simulink model "blown_wing_model"  (R2026a)
settings: Solver=ode23  StopTime=1000  MaxStep=0.05
InitFcn:
  | init_params
values from neighbouring files (symbols this model uses):
  alpha_deg_grid = params.alpha_deg_grid    [init_params.m]
  b = params.b    [init_params.m]
  c = params.c    [init_params.m]    (also in run_aa222_opt.m = clReqProxy - 0.98 * max(params.cl_all_high_lift))
  c_ht = params.c_ht    [init_params.m]
  cd_all_high_lift = params.cd_all_high_lift    [init_params.m]
  cd_blow_only = params.cd_blow_only    [init_params.m]
  cd_clean_baseline = params.cd_clean_baseline    [init_params.m]
  cd_flap_only = params.cd_flap_only    [init_params.m]
  cg_x_m = params.cg_x_m    [init_params.m]
  cl_all_high_lift = params.cl_all_high_lift    [init_params.m]
  CL_alpha_ht = params.CL_alpha_ht    [init_params.m]
  cl_blow_only = params.cl_blow_only    [init_params.m]
  cl_clean_baseline = params.cl_clean_baseline    [init_params.m]
  CL_delta_e = params.CL_delta_e    [init_params.m]
  cl_flap_only = params.cl_flap_only    [init_params.m]
  cm_all_high_lift = params.cm_all_high_lift    [init_params.m]
  cm_blow_only = params.cm_blow_only    [init_params.m]
  cm_clean_baseline = params.cm_clean_baseline    [init_params.m]
  cm_flap_only = params.cm_flap_only    [init_params.m]
  D_prop = params.D_prop    [init_params.m]
  flap_deflection_slow = params.flap_deflection_slow    [init_params.m]
  flap_span_fraction = params.flap_span_fraction    [init_params.m]
  k_span_expansion = params.k_span_expansion    [init_params.m]
  lt = params.lt    [init_params.m]
  params = struct()    [aa222_load_capstone_config.m]    (also in compute_cost.m = aa222_load_capstone_config(fullfile(pwd, 'AA146-Capstone')); init_params.m = aa222_load_capstone_config(capstoneRoot))
  prop_axial_x_m = params.prop_axial_x_m    [init_params.m]
  prop_rpm_grid = params.prop_rpm_grid    [init_params.m]
  prop_thrust_grid = params.prop_thrust_grid    [init_params.m]
  S_ht = params.S_ht    [init_params.m]
  y_dist = params.y_dist    [init_params.m]
libraries: aerolibobsolete x1, aerolibatmos2 x1
settings Model: Creator=olinw  LastModifiedBy=olinw
settings DataIOCC: ExternalInput=utest

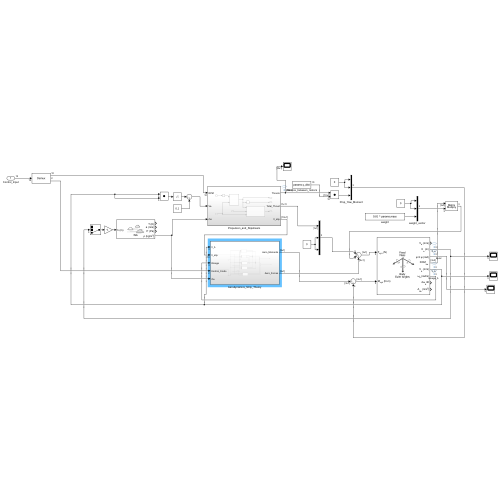
[thumbnail: Simulink's stored preview of the top-level diagram]
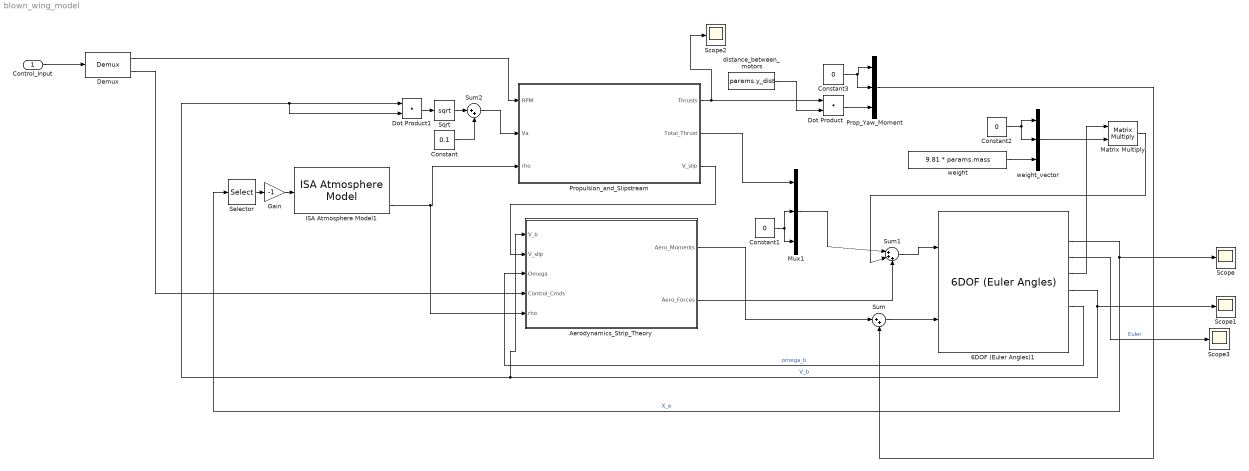
== system blown_wing_model ==
  Control_Input : Inport  PortDimensions=12
  6DOF (Euler Angles)1 : aerolibobsolete/6DOF (Euler Angles)  units=Metric (MKS)  mtype=Fixed  rep=Euler Angles  xme_0=initial_pos_ned  Vm_0=initial_vel_body  eul_0=[0 0 0]  pm_0=[0 0 0]  mass_0=params.mass  mass_e=0.5  mass_f=2.0  inertia=params.InertiaMatrix  inertia_e=eye(3)  inertia_f=2*eye(3)  k_quat=1.0  vre_flag=on  abi_flag=off  aMode=0  xme_statename=''  Vm_statename=''  eul_statename=''  quat_statename=''  pm_statename=''  mass_statename=''
  Aerodynamics_Strip_Theory : Subsystem
  Constant : Constant  Value=0.1
  Constant1 : Constant  Value=0
  Constant2 : Constant  Value=0
  Constant3 : Constant  Value=0
  Demux : Demux  Outputs=[10 2]
      settings: DisplayOption=none
  Dot Product : DotProduct  OutDataTypeStr=Inherit: Inherit via internal rule
  Dot Product1 : DotProduct  OutDataTypeStr=Inherit: Inherit via internal rule
  Gain : Gain  Gain=-1
  ISA Atmosphere Model1 : aerolibatmos2/ISA Atmosphere Model  useExtended=off  action=None  custom=off  viscosityOut=off  g=9.80665  gamma=1.4  R=287.0531  L=0.0065  h_trop=11000  h_strat=20000  rho0=1.225  P0=101325  T0=288.15  h0=0  S=110.4  Tref=273.15  muref=1.716e-5
  Matrix Multiply : Product  Multiplication=Matrix(*)
  Mux1 : Mux  Inputs=3
  Prop_Yaw_Moment : Mux  Inputs=3
  Propulsion_and_Slipstream : Subsystem
  Scope{,1..3} (4 alike) : Scope
      Scope settings: ActiveDisplayYMinimum=-13352.639774194251  ActiveDisplayYMaximum=3591.5339241802285
      Scope1 settings: ActiveDisplayYMinimum=-4.7629764478395824  ActiveDisplayYMaximum=24.22748883276633
      Scope2 settings: ActiveDisplayYMinimum=0.086325999999999986  ActiveDisplayYMaximum=0.28632599999999997  DataLoggingVariableName=ScopeData2
      Scope3 settings: ActiveDisplayYMinimum=-3.92486986686931  ActiveDisplayYMaximum=3.9215936057771783  DataLoggingVariableName=ScopeData3
  Selector : Selector  InputPortWidth=3  IndexOptions=Index vector (dialog)  Indices=3  OutputSizes=1
  Sqrt : Sqrt
  Sum : Sum  Inputs=|++
  Sum1 : Sum  Inputs=|+++
  Sum2 : Sum  Inputs=|++
  distance_between_motors : Constant  Value=params.y_dist
  weight : Constant  Value=9.81 * params.mass
  weight_vector : Mux  Inputs=3
  wires:
  Propulsion_and_Slipstream/2(Total_Thrust) -> Mux1/1
  Constant1/1 -> Mux1/3, Mux1/2
  weight_vector/1 -> Matrix Multiply/2
  Sum1/1 -> 6DOF (Euler Angles)1/1
  6DOF (Euler Angles)1/2 -> Scope/1, Selector/1  "X_e"
  ISA Atmosphere Model1/4 -> Aerodynamics_Strip_Theory/5(rho), Propulsion_and_Slipstream/3(rho)
  6DOF (Euler Angles)1/5 -> Scope1/1, Aerodynamics_Strip_Theory/1(V_b), Dot Product1/2, Dot Product1/1  "V_b"
  Propulsion_and_Slipstream/3(V_slip) -> Aerodynamics_Strip_Theory/2(V_slip)
  Mux1/1 -> Sum1/1
  Aerodynamics_Strip_Theory/2(Aero_Forces) -> Sum1/3
  weight/1 -> weight_vector/3
  distance_between_motors/1 -> Dot Product/2
  Propulsion_and_Slipstream/1(Thrusts) -> Scope2/1, Dot Product/1
  Dot Product/1 -> Prop_Yaw_Moment/3
  Constant3/1 -> Prop_Yaw_Moment/2, Prop_Yaw_Moment/1
  Prop_Yaw_Moment/1 -> Sum/2
  Aerodynamics_Strip_Theory/1(Aero_Moments) -> Sum/1
  Sum/1 -> 6DOF (Euler Angles)1/2
  Constant2/1 -> weight_vector/2, weight_vector/1
  Selector/1 -> Gain/1
  Gain/1 -> ISA Atmosphere Model1/1
  Dot Product1/1 -> Sqrt/1
  Sqrt/1 -> Sum2/1
  Constant/1 -> Sum2/2
  Sum2/1 -> Propulsion_and_Slipstream/2(Va)
  6DOF (Euler Angles)1/4 -> Matrix Multiply/1
  Matrix Multiply/1 -> Sum1/2
  Control_Input/1 -> Demux/1
  6DOF (Euler Angles)1/6 -> Aerodynamics_Strip_Theory/3(Omega)  "omega_b"
  Demux/1 -> Propulsion_and_Slipstream/1(RPM)
  Demux/2 -> Aerodynamics_Strip_Theory/4(Control_Cmds)
  6DOF (Euler Angles)1/3 -> Scope3/1  "Euler"

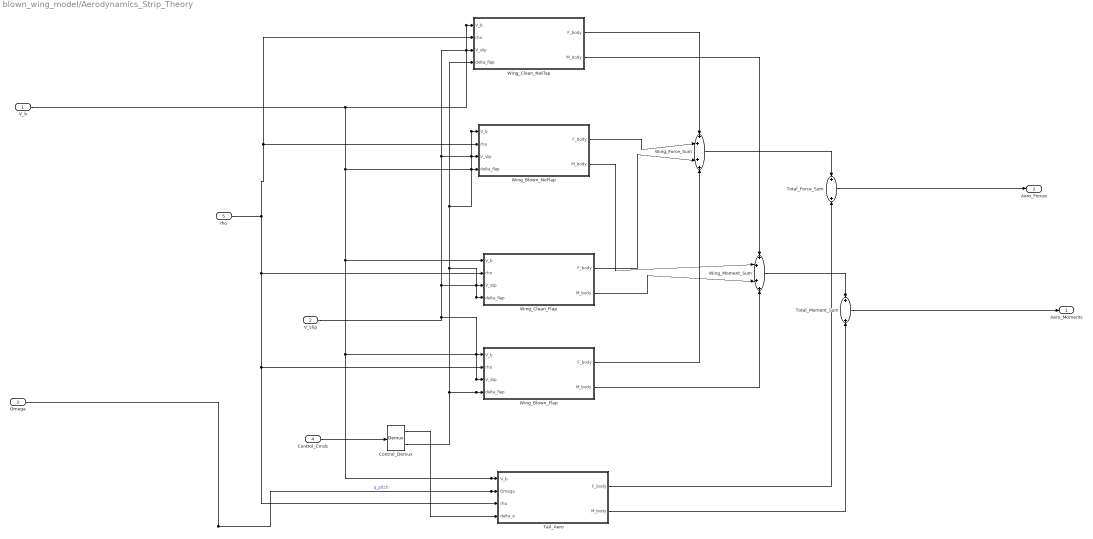
== system blown_wing_model/Aerodynamics_Strip_Theory ==
  V_b : Inport  PortDimensions=3
  V_slip : Inport  Port=2  PortDimensions=10
  Omega : Inport  Port=3
  Control_Cmds : Inport  Port=4
  rho : Inport  Port=5
  Control_Demux : Demux  Outputs=2
  Tail_Aero : Subsystem
  Total_Force_Sum : Sum
  Total_Moment_Sum : Sum
  Wing_Blown_Flap : Subsystem
  Wing_Blown_NoFlap : Subsystem
  Wing_Clean_Flap : Subsystem
  Wing_Clean_NoFlap : Subsystem
  Wing_Force_Sum : Sum  Inputs=++++
  Wing_Moment_Sum : Sum  Inputs=++++
  Aero_Moments : Outport
  Aero_Forces : Outport  Port=2
  wires:
  V_b/1 -> Tail_Aero/1(V_b), Wing_Blown_Flap/1(V_b), Wing_Clean_Flap/1(V_b), Wing_Blown_NoFlap/1(V_b), Wing_Clean_NoFlap/1(V_b)
  V_slip/1 -> Wing_Blown_Flap/3(V_slip), Wing_Blown_NoFlap/3(V_slip), Wing_Clean_NoFlap/3(V_slip), Wing_Clean_Flap/3(V_slip)
  Omega/1 -> Tail_Aero/2(Omega)  "q_pitch"
  Control_Cmds/1 -> Control_Demux/1
  Control_Demux/2 -> Wing_Blown_NoFlap/4(delta_flap), Wing_Clean_NoFlap/4(delta_flap), Wing_Clean_Flap/4(delta_flap), Wing_Blown_Flap/4(delta_flap)
  Control_Demux/1 -> Tail_Aero/4(delta_e)
  Wing_Force_Sum/1 -> Total_Force_Sum/1
  Wing_Moment_Sum/1 -> Total_Moment_Sum/1
  Total_Force_Sum/1 -> Aero_Forces/1
  Total_Moment_Sum/1 -> Aero_Moments/1
  Wing_Clean_NoFlap/1(F_body) -> Wing_Force_Sum/1
  Wing_Clean_NoFlap/2(M_body) -> Wing_Moment_Sum/1
  Wing_Blown_NoFlap/1(F_body) -> Wing_Force_Sum/2
  Wing_Blown_NoFlap/2(M_body) -> Wing_Moment_Sum/2
  Wing_Clean_Flap/1(F_body) -> Wing_Force_Sum/3
  Wing_Clean_Flap/2(M_body) -> Wing_Moment_Sum/3
  Wing_Blown_Flap/1(F_body) -> Wing_Force_Sum/4
  Wing_Blown_Flap/2(M_body) -> Wing_Moment_Sum/4
  Tail_Aero/2(M_body) -> Total_Moment_Sum/2
  Tail_Aero/1(F_body) -> Total_Force_Sum/2
  rho/1 -> Wing_Clean_Flap/2(rho), Tail_Aero/3(rho), Wing_Blown_Flap/2(rho), Wing_Clean_NoFlap/2(rho), Wing_Blown_NoFlap/2(rho)

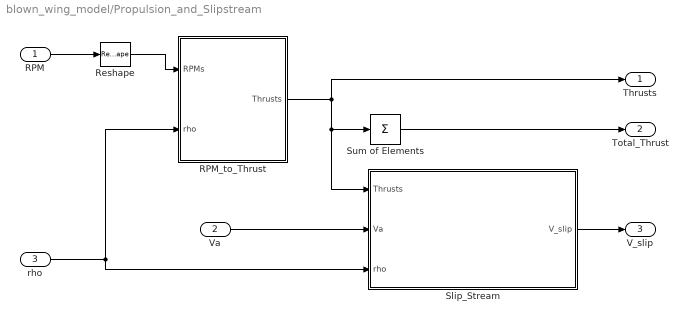
== system blown_wing_model/Propulsion_and_Slipstream ==
  RPM : Inport
  Va : Inport  Port=2
  rho : Inport  Port=3
  RPM_to_Thrust : MATLAB Function  TreatAsAtomicUnit=on
  Reshape : Reshape  OutputDimensionality=Customize  OutputDimensions=[10 1]
  Slip_Stream : MATLAB Function  TreatAsAtomicUnit=on
  Sum of Elements : Sum  Inputs=+
  Thrusts : Outport
  Total_Thrust : Outport  Port=2
  V_slip : Outport  Port=3
  wires:
  RPM_to_Thrust/1(Thrusts) -> Thrusts/1, Slip_Stream/1(Thrusts), Sum of Elements/1
  Sum of Elements/1 -> Total_Thrust/1
  Va/1 -> Slip_Stream/2(Va)
  rho/1 -> RPM_to_Thrust/2(rho), Slip_Stream/3(rho)
  Slip_Stream/1(V_slip) -> V_slip/1
  RPM/1 -> Reshape/1
  Reshape/1 -> RPM_to_Thrust/1(RPMs)

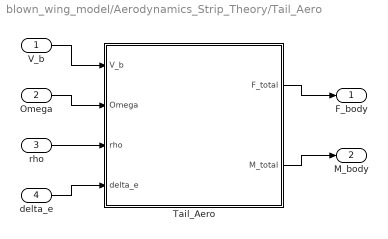
== system blown_wing_model/Aerodynamics_Strip_Theory/Tail_Aero ==
  V_b : Inport
  Omega : Inport  Port=2
  rho : Inport  Port=3
  delta_e : Inport  Port=4
  Tail_Aero : MATLAB Function  TreatAsAtomicUnit=on
  F_body : Outport
  M_body : Outport  Port=2
  wires:
  V_b/1 -> Tail_Aero/1(V_b)
  Omega/1 -> Tail_Aero/2(Omega)
  rho/1 -> Tail_Aero/3(rho)
  delta_e/1 -> Tail_Aero/4(delta_e)
  Tail_Aero/1(F_total) -> F_body/1
  Tail_Aero/2(M_total) -> M_body/1

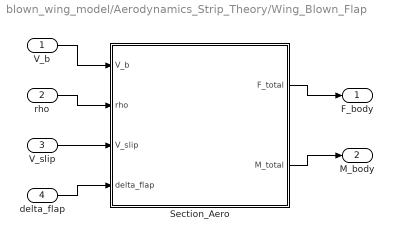
== system blown_wing_model/Aerodynamics_Strip_Theory/Wing_Blown_Flap ==
  V_b : Inport
  rho : Inport  Port=2
  V_slip : Inport  Port=3
  delta_flap : Inport  Port=4
  Section_Aero : MATLAB Function  TreatAsAtomicUnit=on
  F_body : Outport
  M_body : Outport  Port=2
  wires:
  V_b/1 -> Section_Aero/1(V_b)
  rho/1 -> Section_Aero/2(rho)
  V_slip/1 -> Section_Aero/3(V_slip)
  delta_flap/1 -> Section_Aero/4(delta_flap)
  Section_Aero/1(F_total) -> F_body/1
  Section_Aero/2(M_total) -> M_body/1

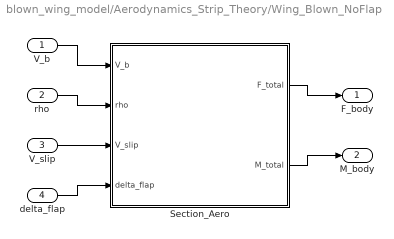
== system blown_wing_model/Aerodynamics_Strip_Theory/Wing_Blown_NoFlap ==
  V_b : Inport
  rho : Inport  Port=2
  V_slip : Inport  Port=3
  delta_flap : Inport  Port=4
  Section_Aero : MATLAB Function  TreatAsAtomicUnit=on
  F_body : Outport
  M_body : Outport  Port=2
  wires:
  V_b/1 -> Section_Aero/1(V_b)
  rho/1 -> Section_Aero/2(rho)
  V_slip/1 -> Section_Aero/3(V_slip)
  delta_flap/1 -> Section_Aero/4(delta_flap)
  Section_Aero/1(F_total) -> F_body/1
  Section_Aero/2(M_total) -> M_body/1

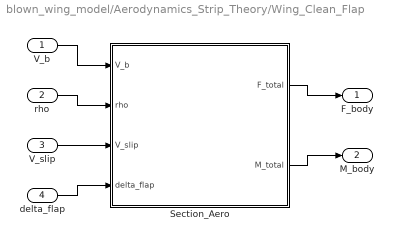
== system blown_wing_model/Aerodynamics_Strip_Theory/Wing_Clean_Flap ==
  V_b : Inport
  rho : Inport  Port=2
  V_slip : Inport  Port=3
  delta_flap : Inport  Port=4
  Section_Aero : MATLAB Function  TreatAsAtomicUnit=on
  F_body : Outport
  M_body : Outport  Port=2
  wires:
  V_b/1 -> Section_Aero/1(V_b)
  rho/1 -> Section_Aero/2(rho)
  V_slip/1 -> Section_Aero/3(V_slip)
  delta_flap/1 -> Section_Aero/4(delta_flap)
  Section_Aero/1(F_total) -> F_body/1
  Section_Aero/2(M_total) -> M_body/1

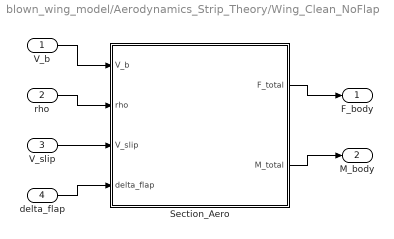
== system blown_wing_model/Aerodynamics_Strip_Theory/Wing_Clean_NoFlap ==
  V_b : Inport
  rho : Inport  Port=2
  V_slip : Inport  Port=3
  delta_flap : Inport  Port=4
  Section_Aero : MATLAB Function  TreatAsAtomicUnit=on
  F_body : Outport
  M_body : Outport  Port=2
  wires:
  V_b/1 -> Section_Aero/1(V_b)
  rho/1 -> Section_Aero/2(rho)
  V_slip/1 -> Section_Aero/3(V_slip)
  delta_flap/1 -> Section_Aero/4(delta_flap)
  Section_Aero/1(F_total) -> F_body/1
  Section_Aero/2(M_total) -> M_body/1

== matlab function blown_wing_model/Aerodynamics_Strip_Theory/Wing_Clean_Flap/Section_Aero ==
  data: V_b input; F_total output; rho input; V_slip input; delta_flap input; M_total output; y_dist parameter; D_prop parameter; b parameter; c parameter; cg_x_m parameter; prop_axial_x_m parameter; flap_span_fraction parameter; flap_deflection_slow parameter; k_span_expansion parameter; alpha_deg_grid parameter; cl_clean_baseline parameter; cl_blow_only parameter; cl_flap_only parameter; cl_all_high_lift parameter; cd_clean_baseline parameter; cd_blow_only parameter; cd_flap_only parameter; cd_all_high_lift parameter; cm_clean_baseline parameter; cm_blow_only parameter; cm_flap_only parameter; cm_all_high_lift parameter
function [F_total, M_total] = Section_Aero(V_b, rho, V_slip, delta_flap, y_dist, D_prop, b, c, cg_x_m, prop_axial_x_m, flap_span_fraction, flap_deflection_slow, k_span_expansion, alpha_deg_grid, cl_clean_baseline, cl_blow_only, cl_flap_only, cl_all_high_lift, cd_clean_baseline, cd_blow_only, cd_flap_only, cd_all_high_lift, cm_clean_baseline, cm_blow_only, cm_flap_only, cm_all_high_lift)
wantBlown = 0;
wantFlap = 1;
F_total = zeros(3,1);
M_total = zeros(3,1);
Vb = reshape(V_b, 3, 1);
Vsl = V_slip(:);
u = Vb(1);
w = Vb(3);
Va = sqrt(sum(Vb.^2)) + 1.0e-3;
alpha = atan2(w, u);
alphaDeg = alpha * 180.0 / pi;
qInf = 0.5 * rho * Va^2;
posMask = y_dist(:) > 0;
posCenters = y_dist(posMask);
posSlip = Vsl(posMask);
blownHalfWidth = 0.5 * k_span_expansion * D_prop;
semiSpan = 0.5 * b;
flapEnd = flap_span_fraction * semiSpan;
edgeList = [0; flapEnd; semiSpan; max(posCenters - blownHalfWidth, 0); min(posCenters + blownHalfWidth, semiSpan)];
edgeList = sort(unique(edgeList));
flapMix = min(max(abs(delta_flap) / max(flap_deflection_slow, 1.0e-6), 0), 1);
ca = cos(alpha);
sa = sin(alpha);
Rsb = [ca, 0, -sa; 0, 1, 0; sa, 0, ca];
for i = 1:(numel(edgeList) - 1)
    y0 = edgeList(i);
    y1 = edgeList(i + 1);
    width = y1 - y0;
    if width <= 1.0e-6
        continue;
    end
    yMid = 0.5 * (y0 + y1);
    isFlapRegion = (yMid <= flapEnd + 1.0e-9);
    overlapMask = (posCenters + blownHalfWidth > y0) & (posCenters - blownHalfWidth < y1);
    isBlownRegion = any(overlapMask);
    if isFlapRegion ~= wantFlap || isBlownRegion ~= wantBlown
        continue;
    end
    qLocal = qInf;
    if isBlownRegion
        vLocal = mean(posSlip(overlapMask));
        qLocal = 0.5 * rho * vLocal^2;
    end
    if wantBlown
        clNoFlap = interp1(alpha_deg_grid, cl_blow_only, alphaDeg, 'linear', 'extrap');
        cdNoFlap = interp1(alpha_deg_grid, cd_blow_only, alphaDeg, 'linear', 'extrap');
        cmNoFlap = interp1(alpha_deg_grid, cm_blow_only, alphaDeg, 'linear', 'extrap');
        clFlap = interp1(alpha_deg_grid, cl_all_high_lift, alphaDeg, 'linear', 'extrap');
        cdFlap = interp1(alpha_deg_grid, cd_all_high_lift, alphaDeg, 'linear', 'extrap');
        cmFlap = interp1(alpha_deg_grid, cm_all_high_lift, alphaDeg, 'linear', 'extrap');
    else
        clNoFlap = interp1(alpha_deg_grid, cl_clean_baseline, alphaDeg, 'linear', 'extrap');
        cdNoFlap = interp1(alpha_deg_grid, cd_clean_baseline, alphaDeg, 'linear', 'extrap');
        cmNoFlap = interp1(alpha_deg_grid, cm_clean_baseline, alphaDeg, 'linear', 'extrap');
        clFlap = interp1(alpha_deg_grid, cl_flap_only, alphaDeg, 'linear', 'extrap');
        cdFlap = interp1(alpha_deg_grid, cd_flap_only, alphaDeg, 'linear', 'extrap');
        cmFlap = interp1(alpha_deg_grid, cm_flap_only, alphaDeg, 'linear', 'extrap');
    end
    if wantFlap
        CL = clNoFlap + flapMix * (clFlap - clNoFlap);
        CD = cdNoFlap + flapMix * (cdFlap - cdNoFlap);
        Cm = cmNoFlap + flapMix * (cmFlap - cmNoFlap);
    else
        CL = clNoFlap;
        CD = cdNoFlap;
        Cm = cmNoFlap;
    end
    areaStrip = c * width;
    Fstab = qLocal * areaStrip * [-CD; 0; -CL];
    Fbody = Rsb * Fstab;
    Maero = qLocal * areaStrip * [0; Cm * c; 0];
    y = yMid;
    rVec = [prop_axial_x_m - cg_x_m; y; 0];
    Mlever = cross(rVec, Fbody);
    F_total = F_total + Fbody;
    M_total = M_total + Maero + Mlever;
    y = -yMid;
    rVec = [prop_axial_x_m - cg_x_m; y; 0];
    Mlever = cross(rVec, Fbody);
    F_total = F_total + Fbody;
    M_total = M_total + Maero + Mlever;
end
end

== matlab function blown_wing_model/Aerodynamics_Strip_Theory/Wing_Blown_Flap/Section_Aero ==
  data: V_b input; F_total output; rho input; V_slip input; delta_flap input; M_total output; y_dist parameter; D_prop parameter; b parameter; c parameter; cg_x_m parameter; prop_axial_x_m parameter; flap_span_fraction parameter; flap_deflection_slow parameter; k_span_expansion parameter; alpha_deg_grid parameter; cl_clean_baseline parameter; cl_blow_only parameter; cl_flap_only parameter; cl_all_high_lift parameter; cd_clean_baseline parameter; cd_blow_only parameter; cd_flap_only parameter; cd_all_high_lift parameter; cm_clean_baseline parameter; cm_blow_only parameter; cm_flap_only parameter; cm_all_high_lift parameter
function [F_total, M_total] = Section_Aero(V_b, rho, V_slip, delta_flap, y_dist, D_prop, b, c, cg_x_m, prop_axial_x_m, flap_span_fraction, flap_deflection_slow, k_span_expansion, alpha_deg_grid, cl_clean_baseline, cl_blow_only, cl_flap_only, cl_all_high_lift, cd_clean_baseline, cd_blow_only, cd_flap_only, cd_all_high_lift, cm_clean_baseline, cm_blow_only, cm_flap_only, cm_all_high_lift)
wantBlown = 1;
wantFlap = 1;
F_total = zeros(3,1);
M_total = zeros(3,1);
Vb = reshape(V_b, 3, 1);
Vsl = V_slip(:);
u = Vb(1);
w = Vb(3);
Va = sqrt(sum(Vb.^2)) + 1.0e-3;
alpha = atan2(w, u);
alphaDeg = alpha * 180.0 / pi;
qInf = 0.5 * rho * Va^2;
posMask = y_dist(:) > 0;
posCenters = y_dist(posMask);
posSlip = Vsl(posMask);
blownHalfWidth = 0.5 * k_span_expansion * D_prop;
semiSpan = 0.5 * b;
flapEnd = flap_span_fraction * semiSpan;
edgeList = [0; flapEnd; semiSpan; max(posCenters - blownHalfWidth, 0); min(posCenters + blownHalfWidth, semiSpan)];
edgeList = sort(unique(edgeList));
flapMix = min(max(abs(delta_flap) / max(flap_deflection_slow, 1.0e-6), 0), 1);
ca = cos(alpha);
sa = sin(alpha);
Rsb = [ca, 0, -sa; 0, 1, 0; sa, 0, ca];
for i = 1:(numel(edgeList) - 1)
    y0 = edgeList(i);
    y1 = edgeList(i + 1);
    width = y1 - y0;
    if width <= 1.0e-6
        continue;
    end
    yMid = 0.5 * (y0 + y1);
    isFlapRegion = (yMid <= flapEnd + 1.0e-9);
    overlapMask = (posCenters + blownHalfWidth > y0) & (posCenters - blownHalfWidth < y1);
    isBlownRegion = any(overlapMask);
    if isFlapRegion ~= wantFlap || isBlownRegion ~= wantBlown
        continue;
    end
    qLocal = qInf;
    if isBlownRegion
        vLocal = mean(posSlip(overlapMask));
        qLocal = 0.5 * rho * vLocal^2;
    end
    if wantBlown
        clNoFlap = interp1(alpha_deg_grid, cl_blow_only, alphaDeg, 'linear', 'extrap');
        cdNoFlap = interp1(alpha_deg_grid, cd_blow_only, alphaDeg, 'linear', 'extrap');
        cmNoFlap = interp1(alpha_deg_grid, cm_blow_only, alphaDeg, 'linear', 'extrap');
        clFlap = interp1(alpha_deg_grid, cl_all_high_lift, alphaDeg, 'linear', 'extrap');
        cdFlap = interp1(alpha_deg_grid, cd_all_high_lift, alphaDeg, 'linear', 'extrap');
        cmFlap = interp1(alpha_deg_grid, cm_all_high_lift, alphaDeg, 'linear', 'extrap');
    else
        clNoFlap = interp1(alpha_deg_grid, cl_clean_baseline, alphaDeg, 'linear', 'extrap');
        cdNoFlap = interp1(alpha_deg_grid, cd_clean_baseline, alphaDeg, 'linear', 'extrap');
        cmNoFlap = interp1(alpha_deg_grid, cm_clean_baseline, alphaDeg, 'linear', 'extrap');
        clFlap = interp1(alpha_deg_grid, cl_flap_only, alphaDeg, 'linear', 'extrap');
        cdFlap = interp1(alpha_deg_grid, cd_flap_only, alphaDeg, 'linear', 'extrap');
        cmFlap = interp1(alpha_deg_grid, cm_flap_only, alphaDeg, 'linear', 'extrap');
    end
    if wantFlap
        CL = clNoFlap + flapMix * (clFlap - clNoFlap);
        CD = cdNoFlap + flapMix * (cdFlap - cdNoFlap);
        Cm = cmNoFlap + flapMix * (cmFlap - cmNoFlap);
    else
        CL = clNoFlap;
        CD = cdNoFlap;
        Cm = cmNoFlap;
    end
    areaStrip = c * width;
    Fstab = qLocal * areaStrip * [-CD; 0; -CL];
    Fbody = Rsb * Fstab;
    Maero = qLocal * areaStrip * [0; Cm * c; 0];
    y = yMid;
    rVec = [prop_axial_x_m - cg_x_m; y; 0];
    Mlever = cross(rVec, Fbody);
    F_total = F_total + Fbody;
    M_total = M_total + Maero + Mlever;
    y = -yMid;
    rVec = [prop_axial_x_m - cg_x_m; y; 0];
    Mlever = cross(rVec, Fbody);
    F_total = F_total + Fbody;
    M_total = M_total + Maero + Mlever;
end
end

== matlab function blown_wing_model/Aerodynamics_Strip_Theory/Tail_Aero/Tail_Aero ==
  data: V_b input; F_total output; Omega input; rho input; delta_e input; M_total output; lt parameter; S_ht parameter; c_ht parameter; CL_alpha_ht parameter; CL_delta_e parameter
function [F_total, M_total] = Tail_Aero(V_b, Omega, rho, delta_e, lt, S_ht, c_ht, CL_alpha_ht, CL_delta_e)
F_total = zeros(3,1);
M_total = zeros(3,1);
Vb = reshape(V_b, 3, 1);
Wb = reshape(Omega, 3, 1);
rTail = [-lt; 0; 0];
Vtail = Vb + cross(Wb, rTail);
u_t = Vtail(1);
w_t = Vtail(3);
Va_t = sqrt(sum(Vtail.^2)) + 0.1;
alpha_t = atan2(w_t, u_t);
qTail = 0.5 * rho * Va_t^2;
CL = CL_alpha_ht * alpha_t + CL_delta_e * delta_e;
CD = 0.02 + 0.06 * CL^2;
Cm = -0.15 * delta_e;
ca = cos(alpha_t);
sa = sin(alpha_t);
Rsb = [ca, 0, -sa; 0, 1, 0; sa, 0, ca];
Fstab = qTail * S_ht * [-CD; 0; -CL];
Fbody = Rsb * Fstab;
Mbody = qTail * S_ht * [0; Cm * c_ht; 0] + cross(rTail, Fbody);
F_total = Fbody;
M_total = Mbody;
end

== matlab function blown_wing_model/Propulsion_and_Slipstream/Slip_Stream ==
  data: Thrusts input; V_slip output; Va input; rho input; D_prop parameter
function V_slip = slipstream_calc(Thrusts, Va, rho, D_prop)
A_prop = pi * (D_prop / 2)^2;
rho_safe = max(rho, 0.1);
T_safe = max(Thrusts, 0);
V_slip = sqrt(max(Va, 0)^2 + (2 .* T_safe) ./ max(rho_safe * A_prop, 1.0e-9));
end

== matlab function blown_wing_model/Propulsion_and_Slipstream/RPM_to_Thrust ==
  data: RPMs input; Thrusts output; rho input; prop_rpm_grid parameter; prop_thrust_grid parameter
function Thrusts = RPM_to_Thrust(RPMs, rho, prop_rpm_grid, prop_thrust_grid)
rpmGrid = prop_rpm_grid(:);
thrustGrid = prop_thrust_grid(:);
Thrusts = zeros(size(RPMs));
for i = 1:numel(RPMs)
    rpm = min(max(RPMs(i), rpmGrid(1)), rpmGrid(end));
    Thrusts(i) = max(interp1(rpmGrid, thrustGrid, rpm, 'linear'), 0);
end
end

== matlab function blown_wing_model/Aerodynamics_Strip_Theory/Wing_Clean_NoFlap/Section_Aero ==
  data: V_b input; F_total output; rho input; V_slip input; delta_flap input; M_total output; y_dist parameter; D_prop parameter; b parameter; c parameter; cg_x_m parameter; prop_axial_x_m parameter; flap_span_fraction parameter; flap_deflection_slow parameter; k_span_expansion parameter; alpha_deg_grid parameter; cl_clean_baseline parameter; cl_blow_only parameter; cl_flap_only parameter; cl_all_high_lift parameter; cd_clean_baseline parameter; cd_blow_only parameter; cd_flap_only parameter; cd_all_high_lift parameter; cm_clean_baseline parameter; cm_blow_only parameter; cm_flap_only parameter; cm_all_high_lift parameter
function [F_total, M_total] = Section_Aero(V_b, rho, V_slip, delta_flap, y_dist, D_prop, b, c, cg_x_m, prop_axial_x_m, flap_span_fraction, flap_deflection_slow, k_span_expansion, alpha_deg_grid, cl_clean_baseline, cl_blow_only, cl_flap_only, cl_all_high_lift, cd_clean_baseline, cd_blow_only, cd_flap_only, cd_all_high_lift, cm_clean_baseline, cm_blow_only, cm_flap_only, cm_all_high_lift)
wantBlown = 0;
wantFlap = 0;
F_total = zeros(3,1);
M_total = zeros(3,1);
Vb = reshape(V_b, 3, 1);
Vsl = V_slip(:);
u = Vb(1);
w = Vb(3);
Va = sqrt(sum(Vb.^2)) + 1.0e-3;
alpha = atan2(w, u);
alphaDeg = alpha * 180.0 / pi;
qInf = 0.5 * rho * Va^2;
posMask = y_dist(:) > 0;
posCenters = y_dist(posMask);
posSlip = Vsl(posMask);
blownHalfWidth = 0.5 * k_span_expansion * D_prop;
semiSpan = 0.5 * b;
flapEnd = flap_span_fraction * semiSpan;
edgeList = [0; flapEnd; semiSpan; max(posCenters - blownHalfWidth, 0); min(posCenters + blownHalfWidth, semiSpan)];
edgeList = sort(unique(edgeList));
flapMix = min(max(abs(delta_flap) / max(flap_deflection_slow, 1.0e-6), 0), 1);
ca = cos(alpha);
sa = sin(alpha);
Rsb = [ca, 0, -sa; 0, 1, 0; sa, 0, ca];
for i = 1:(numel(edgeList) - 1)
    y0 = edgeList(i);
    y1 = edgeList(i + 1);
    width = y1 - y0;
    if width <= 1.0e-6
        continue;
    end
    yMid = 0.5 * (y0 + y1);
    isFlapRegion = (yMid <= flapEnd + 1.0e-9);
    overlapMask = (posCenters + blownHalfWidth > y0) & (posCenters - blownHalfWidth < y1);
    isBlownRegion = any(overlapMask);
    if isFlapRegion ~= wantFlap || isBlownRegion ~= wantBlown
        continue;
    end
    qLocal = qInf;
    if isBlownRegion
        vLocal = mean(posSlip(overlapMask));
        qLocal = 0.5 * rho * vLocal^2;
    end
    if wantBlown
        clNoFlap = interp1(alpha_deg_grid, cl_blow_only, alphaDeg, 'linear', 'extrap');
        cdNoFlap = interp1(alpha_deg_grid, cd_blow_only, alphaDeg, 'linear', 'extrap');
        cmNoFlap = interp1(alpha_deg_grid, cm_blow_only, alphaDeg, 'linear', 'extrap');
        clFlap = interp1(alpha_deg_grid, cl_all_high_lift, alphaDeg, 'linear', 'extrap');
        cdFlap = interp1(alpha_deg_grid, cd_all_high_lift, alphaDeg, 'linear', 'extrap');
        cmFlap = interp1(alpha_deg_grid, cm_all_high_lift, alphaDeg, 'linear', 'extrap');
    else
        clNoFlap = interp1(alpha_deg_grid, cl_clean_baseline, alphaDeg, 'linear', 'extrap');
        cdNoFlap = interp1(alpha_deg_grid, cd_clean_baseline, alphaDeg, 'linear', 'extrap');
        cmNoFlap = interp1(alpha_deg_grid, cm_clean_baseline, alphaDeg, 'linear', 'extrap');
        clFlap = interp1(alpha_deg_grid, cl_flap_only, alphaDeg, 'linear', 'extrap');
        cdFlap = interp1(alpha_deg_grid, cd_flap_only, alphaDeg, 'linear', 'extrap');
        cmFlap = interp1(alpha_deg_grid, cm_flap_only, alphaDeg, 'linear', 'extrap');
    end
    if wantFlap
        CL = clNoFlap + flapMix * (clFlap - clNoFlap);
        CD = cdNoFlap + flapMix * (cdFlap - cdNoFlap);
        Cm = cmNoFlap + flapMix * (cmFlap - cmNoFlap);
    else
        CL = clNoFlap;
        CD = cdNoFlap;
        Cm = cmNoFlap;
    end
    areaStrip = c * width;
    Fstab = qLocal * areaStrip * [-CD; 0; -CL];
    Fbody = Rsb * Fstab;
    Maero = qLocal * areaStrip * [0; Cm * c; 0];
    y = yMid;
    rVec = [prop_axial_x_m - cg_x_m; y; 0];
    Mlever = cross(rVec, Fbody);
    F_total = F_total + Fbody;
    M_total = M_total + Maero + Mlever;
    y = -yMid;
    rVec = [prop_axial_x_m - cg_x_m; y; 0];
    Mlever = cross(rVec, Fbody);
    F_total = F_total + Fbody;
    M_total = M_total + Maero + Mlever;
end
end

== matlab function blown_wing_model/Aerodynamics_Strip_Theory/Wing_Blown_NoFlap/Section_Aero ==
  data: V_b input; F_total output; rho input; V_slip input; delta_flap input; M_total output; y_dist parameter; D_prop parameter; b parameter; c parameter; cg_x_m parameter; prop_axial_x_m parameter; flap_span_fraction parameter; flap_deflection_slow parameter; k_span_expansion parameter; alpha_deg_grid parameter; cl_clean_baseline parameter; cl_blow_only parameter; cl_flap_only parameter; cl_all_high_lift parameter; cd_clean_baseline parameter; cd_blow_only parameter; cd_flap_only parameter; cd_all_high_lift parameter; cm_clean_baseline parameter; cm_blow_only parameter; cm_flap_only parameter; cm_all_high_lift parameter
function [F_total, M_total] = Section_Aero(V_b, rho, V_slip, delta_flap, y_dist, D_prop, b, c, cg_x_m, prop_axial_x_m, flap_span_fraction, flap_deflection_slow, k_span_expansion, alpha_deg_grid, cl_clean_baseline, cl_blow_only, cl_flap_only, cl_all_high_lift, cd_clean_baseline, cd_blow_only, cd_flap_only, cd_all_high_lift, cm_clean_baseline, cm_blow_only, cm_flap_only, cm_all_high_lift)
wantBlown = 1;
wantFlap = 0;
F_total = zeros(3,1);
M_total = zeros(3,1);
Vb = reshape(V_b, 3, 1);
Vsl = V_slip(:);
u = Vb(1);
w = Vb(3);
Va = sqrt(sum(Vb.^2)) + 1.0e-3;
alpha = atan2(w, u);
alphaDeg = alpha * 180.0 / pi;
qInf = 0.5 * rho * Va^2;
posMask = y_dist(:) > 0;
posCenters = y_dist(posMask);
posSlip = Vsl(posMask);
blownHalfWidth = 0.5 * k_span_expansion * D_prop;
semiSpan = 0.5 * b;
flapEnd = flap_span_fraction * semiSpan;
edgeList = [0; flapEnd; semiSpan; max(posCenters - blownHalfWidth, 0); min(posCenters + blownHalfWidth, semiSpan)];
edgeList = sort(unique(edgeList));
flapMix = min(max(abs(delta_flap) / max(flap_deflection_slow, 1.0e-6), 0), 1);
ca = cos(alpha);
sa = sin(alpha);
Rsb = [ca, 0, -sa; 0, 1, 0; sa, 0, ca];
for i = 1:(numel(edgeList) - 1)
    y0 = edgeList(i);
    y1 = edgeList(i + 1);
    width = y1 - y0;
    if width <= 1.0e-6
        continue;
    end
    yMid = 0.5 * (y0 + y1);
    isFlapRegion = (yMid <= flapEnd + 1.0e-9);
    overlapMask = (posCenters + blownHalfWidth > y0) & (posCenters - blownHalfWidth < y1);
    isBlownRegion = any(overlapMask);
    if isFlapRegion ~= wantFlap || isBlownRegion ~= wantBlown
        continue;
    end
    qLocal = qInf;
    if isBlownRegion
        vLocal = mean(posSlip(overlapMask));
        qLocal = 0.5 * rho * vLocal^2;
    end
    if wantBlown
        clNoFlap = interp1(alpha_deg_grid, cl_blow_only, alphaDeg, 'linear', 'extrap');
        cdNoFlap = interp1(alpha_deg_grid, cd_blow_only, alphaDeg, 'linear', 'extrap');
        cmNoFlap = interp1(alpha_deg_grid, cm_blow_only, alphaDeg, 'linear', 'extrap');
        clFlap = interp1(alpha_deg_grid, cl_all_high_lift, alphaDeg, 'linear', 'extrap');
        cdFlap = interp1(alpha_deg_grid, cd_all_high_lift, alphaDeg, 'linear', 'extrap');
        cmFlap = interp1(alpha_deg_grid, cm_all_high_lift, alphaDeg, 'linear', 'extrap');
    else
        clNoFlap = interp1(alpha_deg_grid, cl_clean_baseline, alphaDeg, 'linear', 'extrap');
        cdNoFlap = interp1(alpha_deg_grid, cd_clean_baseline, alphaDeg, 'linear', 'extrap');
        cmNoFlap = interp1(alpha_deg_grid, cm_clean_baseline, alphaDeg, 'linear', 'extrap');
        clFlap = interp1(alpha_deg_grid, cl_flap_only, alphaDeg, 'linear', 'extrap');
        cdFlap = interp1(alpha_deg_grid, cd_flap_only, alphaDeg, 'linear', 'extrap');
        cmFlap = interp1(alpha_deg_grid, cm_flap_only, alphaDeg, 'linear', 'extrap');
    end
    if wantFlap
        CL = clNoFlap + flapMix * (clFlap - clNoFlap);
        CD = cdNoFlap + flapMix * (cdFlap - cdNoFlap);
        Cm = cmNoFlap + flapMix * (cmFlap - cmNoFlap);
    else
        CL = clNoFlap;
        CD = cdNoFlap;
        Cm = cmNoFlap;
    end
    areaStrip = c * width;
    Fstab = qLocal * areaStrip * [-CD; 0; -CL];
    Fbody = Rsb * Fstab;
    Maero = qLocal * areaStrip * [0; Cm * c; 0];
    y = yMid;
    rVec = [prop_axial_x_m - cg_x_m; y; 0];
    Mlever = cross(rVec, Fbody);
    F_total = F_total + Fbody;
    M_total = M_total + Maero + Mlever;
    y = -yMid;
    rVec = [prop_axial_x_m - cg_x_m; y; 0];
    Mlever = cross(rVec, Fbody);
    F_total = F_total + Fbody;
    M_total = M_total + Maero + Mlever;
end
end
